simulink model "uwb_0_delay_mul"  (R2025a)
settings: Solver=VariableStepAuto  StartTime=0.0  StopTime=5e-6  RelTol=1e-3
undefined symbols (not defined in the file or in its folder): j, PSK
libraries: simulink_extras x2, commrfcorlib x1, commsink2 x1, commdigbbndpm3 x1, commchan3 x1
settings Model: Creator=IWMAI  LastModifiedBy=IWMAI

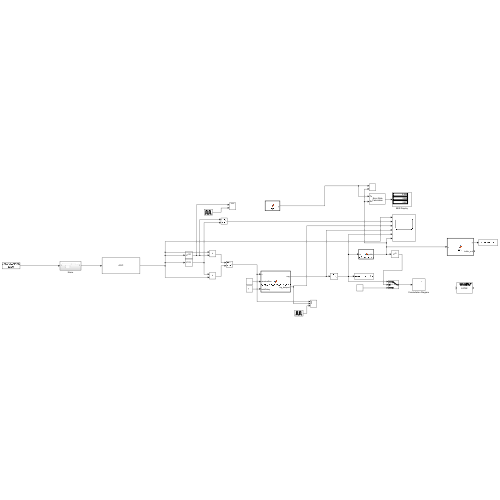
[thumbnail: Simulink's stored preview of the top-level diagram]
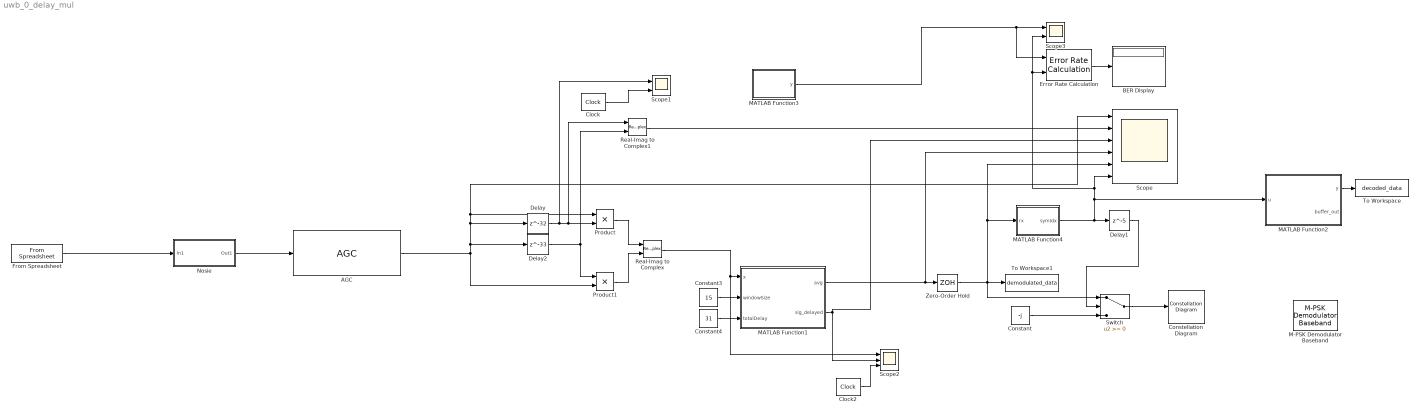
== system uwb_0_delay_mul ==
  AGC : commrfcorlib/AGC  LegacyMode=off  DetectorMethod=Rectifier  LoopMethod=Linear  UpdatePeriod=100  StepSize=0.1  AdaptationStepSize=0.01  DesiredOutputPower=1/2  AveragingLength=100  MaximumGain=30  MaxPowerGain=60  GainOutputPort=off  InputPowerOutputPort=off  SimulateUsing=Interpreted execution
  BER Display : Display
  Clock : simulink_extras/Flip Flops/Clock  period=1/500e6
  Clock2 : simulink_extras/Flip Flops/Clock  period=1/500e6
  Constant : Constant  Value=-j
  Constant3 : Constant  Value=15
  Constant4 : Constant  Value=31
  Constellation Diagram : ConstellationDiagram  WindowPosition=[436.000000,179.000000,986.000000,793.000000,]  Visible=on  ScopeFrameLocation=window  SymbolsToDisplaySource=Property  SymbolsToDisplay=2500  ReferenceConstellation=8-PSK  XLimits=[-2.067197093509777,2.1540515483355467]  YLimits=[-2.067197093509777,2.1540515483355467]  AxesLimits=[-2.067197093509777,2.1540515483355467]  EnableMeasurements=on  DefaultConfigurationName=comm.scopes.ConstellationDiagramBlockCfg
  Delay : Delay  DelayLength=32
  Delay1 : Delay  DelayLength=5  InitialCondition=-1
  Delay2 : Delay  DelayLength=33
  Error Rate Calculation : commsink2/Error Rate Calculation  N=0  st_delay=0  cp_mode=Entire frame  subframe=[]  PMode=Port  WsName=ErrorVec  RsMode2=off  stop=off  numErr=100  maxBits=1e6
      settings: LibrarySourceBlock=|
      | commhdlsink/Error Rate
      | Calculation
  From Spreadsheet : FromSpreadsheet  FileName=C:\Users\IWMAI\University of Toronto\Yu Huang - Summer-2025-sharted\Yongkang\v4_250623\csv\data16.csv  SheetName=data16  SampleTime=1/16e9  ExtrapolationBeforeFirstDataPoint=Hold first value  InterpolationWithinTimeRange=Zero order hold  ExtrapolationAfterLastDataPoint=Hold last value
  M-PSK Demodulator Baseband : commdigbbndpm3/M-PSK Demodulator Baseband  M=8  OutType=Integer  DecType=Hard decision  VarSource=Dialog  Variance=1  Dec=Gray  Mapping=[0:7]  Ph=pi/8  outDtype1=Inherit via internal rule  outDtype2=Inherit via internal rule  derotateFactorWordLen=16  derotateFactorDataTypeStr=Inherit: Same word length as input  derotateFactorLastDataTypeStr=Inherit: Same word length as input
      settings: LibrarySourceBlock=|
      | commhdldigbbndpm/M-PSK
      | Demodulator
      | Baseband
  MATLAB Function1 : MATLAB Function  TreatAsAtomicUnit=on
  MATLAB Function2 : MATLAB Function  TreatAsAtomicUnit=on
  MATLAB Function3 : MATLAB Function  TreatAsAtomicUnit=on  SystemSampleTime=1/500e6
  MATLAB Function4 : MATLAB Function  TreatAsAtomicUnit=on
  Nosie : Subsystem
  Product : Product
  Product1 : Product
  Real-Imag to Complex : RealImagToComplex
  Real-Imag to Complex1 : RealImagToComplex
  Scope : Scope  NumInputPorts=6
      settings: ActiveDisplayYMinimum=-3.4036686172419608  ActiveDisplayYMaximum=3.0401772785290166
  Scope1 : Scope  NumInputPorts=2
      settings: ActiveDisplayYMinimum=-1.2499999999999791  ActiveDisplayYMaximum=1.2499999999999976
  Scope2 : Scope  NumInputPorts=3
      settings: ActiveDisplayYMinimum=-3.0942318111750153  ActiveDisplayYMaximum=3.1921236697728448  DataLoggingVariableName=ScopeData2
  Scope3 : Scope  NumInputPorts=2
      settings: ActiveDisplayYMinimum=-0.69396207709214863  ActiveDisplayYMaximum=8.0560379229078443  DataLoggingVariableName=ScopeData3
  Switch : Switch  SaturateOnIntegerOverflow=off  InputSameDT=off
  To Workspace : ToWorkspace  VariableName=decoded_data  SaveFormat=Structure With Time  SampleTime=-1
  To Workspace1 : ToWorkspace  VariableName=demodulated_data  SaveFormat=Structure With Time  SampleTime=-1
  Zero-Order Hold : ZeroOrderHold  SampleTime=1/500e6
  wires:
  Delay/1 -> Product/2, Real-Imag to Complex1/1, Scope1/1
  Delay2/1 -> Real-Imag to Complex1/2, Product1/1
  Product/1 -> Real-Imag to Complex/1
  Product1/1 -> Real-Imag to Complex/2
  Zero-Order Hold/1 -> To Workspace1/1, Switch/1, MATLAB Function4/1(rx), Scope/5
  MATLAB Function4/1(symIdx) -> Delay1/1, Scope3/2, Error Rate Calculation/2, Scope/6, MATLAB Function2/1(u)
  Real-Imag to Complex1/1 -> Scope/2
  Delay1/1 -> Switch/2
  Switch/1 -> Constellation Diagram/1
  Constant/1 -> Switch/3
  Clock/1 -> Scope1/2
  AGC/1 -> Delay2/1, Delay/1, Scope/1, Product/1, Product1/2
  Constant3/1 -> MATLAB Function1/2(windowSize)
  MATLAB Function1/1(avg) -> Scope/4, Zero-Order Hold/1
  MATLAB Function1/2(sig_delayed) -> Scope/3, Scope2/2
  Constant4/1 -> MATLAB Function1/3(totalDelay)
  Real-Imag to Complex/1 -> MATLAB Function1/1(x), Scope2/1
  Clock2/1 -> Scope2/3
  MATLAB Function2/1(y) -> To Workspace/1
  MATLAB Function3/1(y) -> Error Rate Calculation/1, Scope3/1
  Error Rate Calculation/1 -> BER Display/1
  From Spreadsheet/1 -> Nosie/1(In1)
  Nosie/1(Out1) -> AGC/1

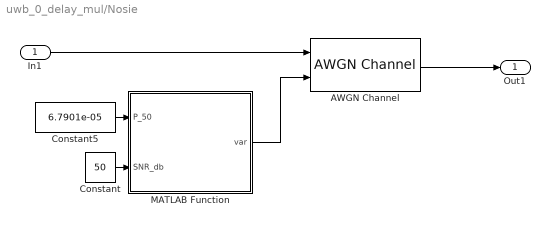
== system uwb_0_delay_mul/Nosie ==
  In1 : Inport
  AWGN Channel : commchan3/AWGN Channel  LegacyMode=off  NoiseMethod=Variance  noiseMode="Signal to noise ratio  (SNR)"  EbNo=10  EsNo=10  SNR=5  BitsPerSymbol=1  SignalPower=1  SpecifySymbolPeriod=off  SamplesPerSymbol=1  SymbolPeriod=1  VarianceSource=Input port  Variance=1  RandomStream=mt19937ar with seed  Seed=67  SimulateUsing=Code generation
  Constant : Constant  Value=50
  Constant5 : Constant  Value=6.7901e-05
  MATLAB Function : MATLAB Function  TreatAsAtomicUnit=on
  Out1 : Outport
  wires:
  In1/1 -> AWGN Channel/1
  AWGN Channel/1 -> Out1/1
  MATLAB Function/1(var) -> AWGN Channel/2
  Constant5/1 -> MATLAB Function/1(P_50)
  Constant/1 -> MATLAB Function/2(SNR_db)

== matlab function uwb_0_delay_mul/MATLAB Function1 ==
  data: x input; avg output; windowSize input; totalDelay input; sig_delayed output
function [avg, sig_delayed] = mov_avg_fixed_delay_even_window(x, windowSize, totalDelay)
% mov_avg_fixed_delay_even_window: Calculates a moving average and the original signal, both with a fixed total delay.
%
%   This version supports even window sizes by rounding the inherent delay.
%
%   Parameters:
%   x:            Input signal (scalar).
%   windowSize:   The size of the moving average window. Must be a positive integer.
%   totalDelay:   The desired total output delay (in samples). Must be an integer.
%
%   Outputs:
%   avg:          The moving average of the signal, delayed by 'totalDelay'.
%   sig_delayed:  The original signal 'x', delayed by 'totalDelay'.

% 1. Persistent variable declaration
persistent avgCalcBuffer;
persistent avgDelayBuffer;
persistent signalDelayBuffer;
persistent avgDelayPtr;
persistent sigDelayPtr;
persistent isInitialized;

% 2. Input Validation & Delay Calculation
if windowSize <= 0
    error('Window size (windowSize) must be a positive integer.');
end

% Calculate inherent delay. For even window sizes, this will be X.5.
% We will round it up to the next integer for buffer management.
inherentDelay_float = (windowSize - 1) / 2;
inherentDelay = ceil(inherentDelay_float); % Round up to the next integer delay

if totalDelay < inherentDelay
    error('Total delay (%d) must be >= inherent moving average delay (%d, rounded up from %.1f).', totalDelay, inherentDelay, inherentDelay_float);
end

additionalDelay = totalDelay - inherentDelay;

% 3. Initialize Buffers (on first call only)
if isempty(isInitialized)
    avgCalcBuffer = zeros(1, windowSize, 'like', x);

    signalDelayBuffer = zeros(1, 0, 'like', x);
    avgDelayBuffer = zeros(1, 0, 'like', x);

    sigDelayPtr = 1;
    avgDelayPtr = 1;

    if totalDelay > 0
        signalDelayBuffer = zeros(1, totalDelay, 'like', x);
    end

    if additionalDelay > 0
        avgDelayBuffer = zeros(1, additionalDelay, 'like', x);
    end

    isInitialized = true;
end

% 4. Update Buffers and Perform Calculations
% --- Step 4a: Update Moving Average Calculation Buffer ---
avgCalcBuffer(1:end-1) = avgCalcBuffer(2:end);
avgCalcBuffer(end) = x;
currentAvg = sum(avgCalcBuffer) / windowSize;

% --- Step 4b: Process the Signal Delay using a circular buffer ---
if totalDelay > 0
    sig_delayed = signalDelayBuffer(sigDelayPtr);
    signalDelayBuffer(sigDelayPtr) = x;
    if sigDelayPtr == totalDelay
        sigDelayPtr = 1;
    else
        sigDelayPtr = sigDelayPtr + 1;
    end
else
    sig_delayed = x;
end

% --- Step 4c: Process the Average Delay using a circular buffer ---
if additionalDelay > 0
    avg = avgDelayBuffer(avgDelayPtr);
    avgDelayBuffer(avgDelayPtr) = currentAvg;
    if avgDelayPtr == additionalDelay
        avgDelayPtr = 1;
    else
        avgDelayPtr = avgDelayPtr + 1;
    end
else
    avg = currentAvg;
end
end

== matlab function uwb_0_delay_mul/Nosie/MATLAB Function ==
  data: P_50 input; var output; SNR_db input
function var = calc_SNR(P_50, SNR_db)

% calculate the variance based on the power of 50 ohm

SNR_linear = 10 ^ (SNR_db / 10);

P_noise_50 = P_50 / SNR_linear;

% P_noise_50 = var ^ 2 / Z
% var ^ 2 = P_noise_50 * 50
var = P_noise_50 * 50;

== matlab function uwb_0_delay_mul/MATLAB Function2 ==
  data: u input; y output; buffer_out output
function [y, buffer_out] = save(u)
% This function stores input 'u' into a persistent buffer.
% 'buf_len' defines the maximum length of the buffer.

persistent buffer; % Declares 'buffer' as a persistent variable
persistent index;  % Declares 'index' as a persistent variable

% Initialize buffer and index if they are empty (first call)
if isempty(buffer)
    buffer = zeros(2500, 1); % Initialize with zeros, make it a column vector
    index = 1; % Start index at 1
end

% Store the input 'u' into the buffer
% Use mod to wrap around the buffer if it's full, or just increment
% For a fixed-size buffer that overwrites, you might use:
% actual_index = mod(index - 1, buf_len) + 1;
% buffer(actual_index) = u;

% If you want to fill the buffer and then stop, or keep filling beyond buf_len (growing buffer)
% For simplicity here, let's assume you want to fill it up to buf_len
if index <= 2500
    buffer(index) = u;
else
    % If buffer is full, you might want to handle it (e.g., overwrite oldest, or stop writing)
    % For this example, let's just keep writing to the last element if index exceeds buf_len
    % or simply stop updating the buffer if it's full and you don't want to overwrite
    % For now, we'll just keep the last value if index goes beyond buf_len,
    % or you could ensure it always points to a valid index by wrapping.
    % To wrap around:
    buffer(mod(index - 1, 2500) + 1) = u;
end

index = index + 1; % Increment the index for the next call

% Output 'y' is the current input 'u' (as in your original code)
y = u;

% 'buffer_out' is the current state of the buffer
% This output will be connected to a To Workspace block
buffer_out = buffer;

end

== matlab function uwb_0_delay_mul/MATLAB Function3 ==
  data: y output
function y = fcn

persistent index;
persistent ans_buffer;

buffer_len = 127;

if isempty(index)
    index = 1;
    ans_buffer = [7 4 2 2 2 2 2 6 5 3 3 3 3 7 2 7 5 5 5 1 0 2 1 7 7 3 6 7 0 5 3 7 6 4 4 0 7 1 4 1 7 3 6 7 4 6 5 7 6 4 0 3 4 5 6 3 5 4 2 2 2 6 1 2 7 5 5 1 0 6 2 1 7 3 6 3 5 0 5 7 6 0 3 0 2 5 6 7 4 6 1 6 4 4 0 3 0 2 1 7 3 2 4 7 0 5 7 2 3 0 6 2 5 2 0 4 3 5 4 6 5 7 2 3 4 5 6];
end

y = ans_buffer(mod(index, buffer_len) + 1);
index = index + 1;

== matlab function uwb_0_delay_mul/MATLAB Function4 ==
  data: rx input; symIdx output
function symIdx = my_8psk_decoder(rx)
% rx: complex input symbol
% symIdx: integer index [0~7]

% 固定参考点（从 Python 得到）
persistent centers
if isempty(centers)
    centers = [
-0.794546 + -0.298444i;
-0.425530 + -0.703649i;
0.731182 + -0.125290i;
0.232761 + -0.730665i;
-0.220880 + 0.731179i;
-0.772253 + 0.362395i;
0.270349 + 0.746917i;
0.682762 + 0.402678i;
    ]; % 改成你实际的
end

% 最小距离判决
dist = abs(rx - centers);
[~, symIdx] = min(dist);

symIdx = symIdx - 1; % MATLAB index从1开始，转成0~7
